simulink model "simscape_trial_simplified"  (R2020a)
settings: Solver=VariableStepAuto  StartTime=0.0  StopTime=tf  FixedStep=0.001  MaxStep=.0001  RelTol=1e-3  AbsTol=1e-3
PreLoadFcn:
  | simscape_trial_simplified_script
undefined symbols (not defined in the file): DC, numberNozzles
libraries: nesl_utility x7, fl_lib x6, SimscapeFluids_lib x6, sh_lib x2
settings Model: Creator=kenny  LastModifiedBy=voncken
settings SolverCC: AutoScaleAbsTol=off
settings DebuggingCC: SymbolicDimsDataTypeCodeGenerationDiagnostic=none
settings SFSimCC: CustomCodeUndefinedFunction=UseInterfaceOnly
settings SimscapeCC: SimscapeLogType=all  SimscapeLogSimulationStatistics=on  SimscapeLogLimitData=off  SimscapeLogDataHistory=10000

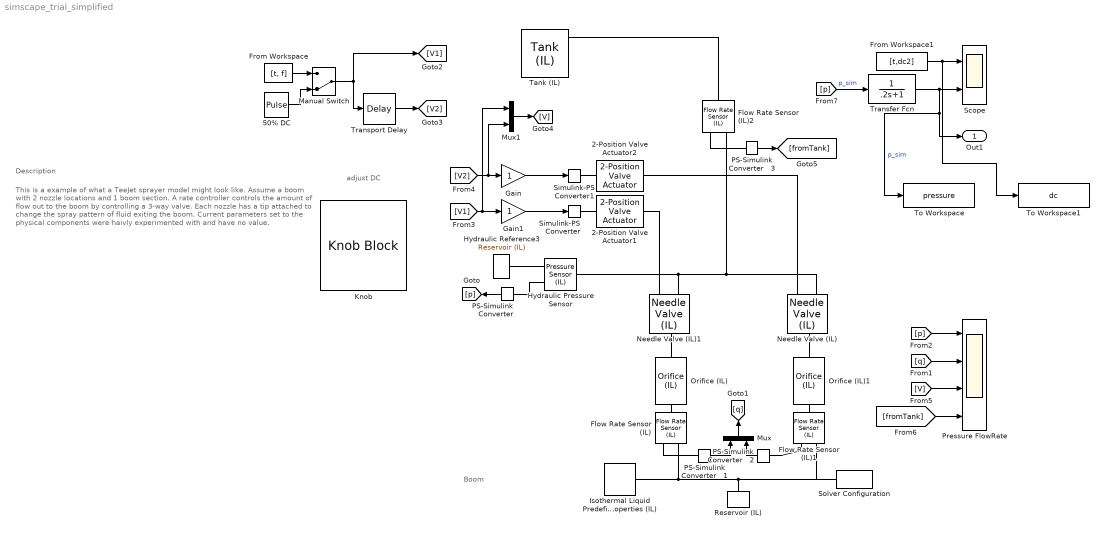
== system simscape_trial_simplified ==
  note: adjust DC
  note: Boom
  note: Description
  note: This is a example of what a TeeJet sprayer model might look like. Assume a boom with 2 nozzle locations and 1 boom section. A rate controller controls the amount of flow out to the boom by controlling a 3-way valve. Each nozzle has a tip attached to change the spray pattern of fluid exiting the boom.
      | Current parameters set to the physical components were haivly experimented with and have no value.
  2-Position Valve Actuator1 : sh_lib/Valves/Valve Actuators/2-Position Valve Actuator  stroke=h_MAX m  t_on=0.002 s  t_off=0.002 s  act_signal=12  init_position=0  act_orientation=1
      settings: SourceProductBaseCode=SH  InternalSimscapePortConfiguration="{\"Bottom\":[],\"Left\":[{\"id\":\"C\",\"label\":\"\",\"type\":\"input\"}],\"Right\":[{\"id\":\"P\",\"label\":\"\",\"type\":\"output\"}],\"Top\":[]}"
  2-Position Valve Actuator2 : sh_lib/Valves/Valve Actuators/2-Position Valve Actuator  stroke=h_MAX m  t_on=0.002 s  t_off=0.002 s  act_signal=12  init_position=0  act_orientation=1
      settings: SourceProductBaseCode=SH  InternalSimscapePortConfiguration="{\"Bottom\":[],\"Left\":[{\"id\":\"C\",\"label\":\"\",\"type\":\"input\"}],\"Right\":[{\"id\":\"P\",\"label\":\"\",\"type\":\"output\"}],\"Top\":[]}"
  "50% DC  " : DiscretePulseGenerator  PulseType=Time based  Amplitude=12  Period=.05  PulseWidth=DC
  Flow Rate Sensor (IL) : fl_lib/Isothermal Liquid/Sensors/Flow Rate Sensor (IL)  sensor_type=foundation.enum.mass_volumetric_sensor.volumetric
      settings: SourceProductBaseCode=SS  InternalSimscapePortConfiguration="{\"Bottom\":[],\"Left\":[{\"id\":\"A\",\"label\":\"A\",\"type\":\"foundation.isothermal_liquid.isothermal_liquid\"}],\"Right\":[{\"id\":\"B\",\"label\":\"B\",\"type\":\"foundation.isothermal_liquid.isothermal_liquid\"},{\"id\":\"V\",\"label\":\"V\",\"type\":\"output\"}],\"Top\":[]}"
  Flow Rate Sensor (IL)1 : fl_lib/Isothermal Liquid/Sensors/Flow Rate Sensor (IL)  sensor_type=foundation.enum.mass_volumetric_sensor.volumetric
      settings: SourceProductBaseCode=SS  InternalSimscapePortConfiguration="{\"Bottom\":[],\"Left\":[{\"id\":\"A\",\"label\":\"A\",\"type\":\"foundation.isothermal_liquid.isothermal_liquid\"}],\"Right\":[{\"id\":\"B\",\"label\":\"B\",\"type\":\"foundation.isothermal_liquid.isothermal_liquid\"},{\"id\":\"V\",\"label\":\"V\",\"type\":\"output\"}],\"Top\":[]}"
  Flow Rate Sensor (IL)2 : fl_lib/Isothermal Liquid/Sensors/Flow Rate Sensor (IL)  sensor_type=foundation.enum.mass_volumetric_sensor.volumetric
      settings: SourceProductBaseCode=SS  InternalSimscapePortConfiguration="{\"Bottom\":[],\"Left\":[{\"id\":\"A\",\"label\":\"A\",\"type\":\"foundation.isothermal_liquid.isothermal_liquid\"}],\"Right\":[{\"id\":\"B\",\"label\":\"B\",\"type\":\"foundation.isothermal_liquid.isothermal_liquid\"},{\"id\":\"V\",\"label\":\"V\",\"type\":\"output\"}],\"Top\":[]}"
  From Workspace : FromWorkspace  VariableName=[t, f]
  From Workspace1 : FromWorkspace  VariableName=[t,dc2]  SampleTime=-1
  Gain : Gain
  Gain1 : Gain
  Hydraulic Pressure Sensor : fl_lib/Isothermal Liquid/Sensors/Pressure Sensor (IL)  pressure_measure=foundation.enum.pressure_measure.difference
      settings: SourceProductBaseCode=SS  InternalSimscapePortConfiguration="{\"Bottom\":[],\"Left\":[{\"id\":\"A\",\"label\":\"A\",\"type\":\"foundation.isothermal_liquid.isothermal_liquid\"}],\"Right\":[{\"id\":\"B\",\"label\":\"B\",\"type\":\"foundation.isothermal_liquid.isothermal_liquid\"},{\"id\":\"P\",\"label\":\"P\",\"type\":\"output\"}],\"Top\":[]}"
  Hydraulic Reference3 : fl_lib/Isothermal Liquid/Elements/Reservoir (IL)  reservoir_type=foundation.enum.constant_controlled.constant  pressure_spec=foundation.enum.pressure_spec.atmospheric  reservoir_pressure=0.101325 MPa
      settings: SourceProductBaseCode=SS
  Isothermal Liquid Predefined Properties (IL) : SimscapeFluids_lib/Isothermal Liquid/Utilities/Isothermal Liquid Predefined Properties (IL)  fluid_list=fluids.isothermal_liquid.utilities.enum.isothermal_liquid_fluid_list.water  concentration_param_EG=fluids.isothermal_liquid.utilities.enum.isothermal_liquid_concentration.volume_fraction  concentration_param_PG=fluids.isothermal_liquid.utilities.enum.isothermal_liquid_concentration.volume_fraction  c_mass_SW=3.5e-3  c_mass_EG=0.1  c_mass_PG=0.1  c_mass_GL=0.1  c_vol_EG=0.1  c_vol_PG=0.1  beta_L_atm_EG=2.1791 GPa  beta_L_atm_PG=2.1791 GPa  beta_L_atm_GL=2.1791 GPa  p_min_EG=0.01 MPa  p_min_PG=0.01 MPa  p_min_GL=0.01 MPa  T=293.15 K  air_fraction=0  polytropic_index=1.0  rho_g_atm=1.225 kg/m^3  air_dissolution_model=simscape.enum.onoff.off  p_crit=3 MPa  derate_coeff=1  p_atm=0.101325 MPa
      settings: SourceProductBaseCode=SH  InternalSimscapePortConfiguration="{\"Bottom\":[],\"Left\":[],\"Right\":[{\"id\":\"A\",\"label\":\"\",\"type\":\"foundation.isothermal_liquid.isothermal_liquid\"}],\"Top\":[]}"
  Knob : KnobBlock  TickInterval=10
  Manual Switch : ManualSwitch  CurrentSetting=0
  Mux : Mux  Inputs=2
  Mux1 : Mux  Inputs=2
  Needle Valve (IL) : SimscapeFluids_lib/Isothermal Liquid/Valves & Orifices/Flow Control Valves/Needle Valve (IL)  diam_orifice=5e-3 m  cone_angle=90 deg  S_min=0 m  area_leak=1e-10*numberNozzles m^2  area=inf m^2  Cd=0.64  Re_c=150  pressure_recovery=simscape.enum.onoff.off  mdot_A_specify=off  mdot_A_priority=None  mdot_A=0 kg/s  mdot_A_nominal_specify=off  mdot_A_nominal_unit=kg/s  mdot_A_nominal_value=1  mdot_B_specify=off  mdot_B_priority=None  mdot_B=0 kg/s  mdot_B_nominal_specify=off  mdot_B_nominal_unit=kg/s  mdot_B_nominal_value=1
      settings: SourceProductBaseCode=SH  InternalSimscapePortConfiguration="{\"Bottom\":[],\"Left\":[{\"id\":\"A\",\"label\":\"A\",\"type\":\"foundation.isothermal_liquid.isothermal_liquid\"},{\"id\":\"S\",\"label\":\"S\",\"type\":\"input\"}],\"Right\":[{\"id\":\"B\",\"label\":\"B\",\"type\":\"foundation.isothermal_liquid.isothermal_liquid\"}],\"Top\":[]}"
  Needle Valve (IL)1 : SimscapeFluids_lib/Isothermal Liquid/Valves & Orifices/Flow Control Valves/Needle Valve (IL)  diam_orifice=d_0 m  cone_angle=theta rad  S_min=0 m  area_leak=1e-10*numberNozzles m^2  area=inf m^2  Cd=0.64  Re_c=150  pressure_recovery=simscape.enum.onoff.off  mdot_A_specify=off  mdot_A_priority=None  mdot_A=0 kg/s  mdot_A_nominal_specify=off  mdot_A_nominal_unit=kg/s  mdot_A_nominal_value=1  mdot_B_specify=off  mdot_B_priority=None  mdot_B=0 kg/s  mdot_B_nominal_specify=off  mdot_B_nominal_unit=kg/s  mdot_B_nominal_value=1
      settings: SourceProductBaseCode=SH  InternalSimscapePortConfiguration="{\"Bottom\":[],\"Left\":[{\"id\":\"A\",\"label\":\"A\",\"type\":\"foundation.isothermal_liquid.isothermal_liquid\"},{\"id\":\"S\",\"label\":\"S\",\"type\":\"input\"}],\"Right\":[{\"id\":\"B\",\"label\":\"B\",\"type\":\"foundation.isothermal_liquid.isothermal_liquid\"}],\"Top\":[]}"
  Orifice (IL) : SimscapeFluids_lib/Isothermal Liquid/Valves & Orifices/Orifices/Orifice (IL)  orifice_type=foundation.enum.constant_variable.constant  constant_orifice_spec=fluids.isothermal_liquid.valves_orifices.orifices.enum.constant_orifice_spec.table1D_volflow_pressure  variable_orifice_spec=fluids.isothermal_liquid.valves_orifices.orifices.enum.orifice_spec.linear  orifice_area_constant=1e-3 m^2  p_diff_TLU_constant=pressureDrop psi  vol_flow_TLU_constant=volFlowRate gpm  S_min=0 m  del_S=5e-3 m  open_orientation=fluids.isothermal_liquid.valves_orifices.orifices.enum.orifice_orientation.positive  area_max=1e-4 m^2  area_leak=1e-10 m^2  S_TLU=[0, .002, .004, .007, .017] m  orifice_area_TLU=[1e-09, 2.0352e-07, 4.0736e-05, .00011438, .00034356] m^2  area=inf m^2  Cd=0.64  Re_c=150  pressure_recovery=simscape.enum.onoff.off  S_vol_flow_TLU=[0, .002, .004, .007, .017] m  p_diff_TLU=[.3, .5, .7] MPa  vol_flow_TLU=1e-3 * [1.7e-05, 2e-05, 2.6e-05; .0035, .0045, .0053; .7, .9, 1.06; 1.96, 2.5, 3; 6, 7.7, 9.13] m^3/s  mdot_A_specify=off  mdot_A_priority=None  mdot_A=0 kg/s  mdot_A_nominal_specify=off  mdot_A_nominal_unit=kg/s  mdot_A_nominal_value=1  mdot_B_specify=off  mdot_B_priority=None  mdot_B=0 kg/s  mdot_B_nominal_specify=off  mdot_B_nominal_unit=kg/s  mdot_B_nominal_value=1
      settings: SourceProductBaseCode=SH  InternalSimscapePortConfiguration="{\"Bottom\":[],\"Left\":[{\"id\":\"A\",\"label\":\"A\",\"type\":\"foundation.isothermal_liquid.isothermal_liquid\"}],\"Right\":[{\"id\":\"B\",\"label\":\"B\",\"type\":\"foundation.isothermal_liquid.isothermal_liquid\"}],\"Top\":[]}"
  Orifice (IL)1 : SimscapeFluids_lib/Isothermal Liquid/Valves & Orifices/Orifices/Orifice (IL)  orifice_type=foundation.enum.constant_variable.constant  constant_orifice_spec=fluids.isothermal_liquid.valves_orifices.orifices.enum.constant_orifice_spec.table1D_volflow_pressure  variable_orifice_spec=fluids.isothermal_liquid.valves_orifices.orifices.enum.orifice_spec.linear  orifice_area_constant=1e-3 m^2  p_diff_TLU_constant=pressureDrop psi  vol_flow_TLU_constant=volFlowRate gpm  S_min=0 m  del_S=5e-3 m  open_orientation=fluids.isothermal_liquid.valves_orifices.orifices.enum.orifice_orientation.positive  area_max=1e-4 m^2  area_leak=1e-10 m^2  S_TLU=[0, .002, .004, .007, .017] m  orifice_area_TLU=[1e-09, 2.0352e-07, 4.0736e-05, .00011438, .00034356] m^2  area=inf m^2  Cd=0.64  Re_c=150  pressure_recovery=simscape.enum.onoff.off  S_vol_flow_TLU=[0, .002, .004, .007, .017] m  p_diff_TLU=[.3, .5, .7] MPa  vol_flow_TLU=1e-3 * [1.7e-05, 2e-05, 2.6e-05; .0035, .0045, .0053; .7, .9, 1.06; 1.96, 2.5, 3; 6, 7.7, 9.13] m^3/s  mdot_A_specify=off  mdot_A_priority=None  mdot_A=0 kg/s  mdot_A_nominal_specify=off  mdot_A_nominal_unit=kg/s  mdot_A_nominal_value=1  mdot_B_specify=off  mdot_B_priority=None  mdot_B=0 kg/s  mdot_B_nominal_specify=off  mdot_B_nominal_unit=kg/s  mdot_B_nominal_value=1
      settings: SourceProductBaseCode=SH  InternalSimscapePortConfiguration="{\"Bottom\":[],\"Left\":[{\"id\":\"A\",\"label\":\"A\",\"type\":\"foundation.isothermal_liquid.isothermal_liquid\"}],\"Right\":[{\"id\":\"B\",\"label\":\"B\",\"type\":\"foundation.isothermal_liquid.isothermal_liquid\"}],\"Top\":[]}"
  "PS-Simulink Converter   " : nesl_utility/PS-Simulink Converter  PhysicalDomain=network_engine_domain  SubClassName=ps_output  LeftPortType=input  RightPortType=output  PseudoPeriodic=off  Frequencies=[]  Unit=bar  AffineConversion=off
      settings: SourceProductBaseCode=MT,SS
  PS-Simulink Converter   1 : nesl_utility/PS-Simulink Converter  PhysicalDomain=network_engine_domain  SubClassName=ps_output  LeftPortType=input  RightPortType=output  PseudoPeriodic=off  Frequencies=[]  Unit=gpm  AffineConversion=off
      settings: SourceProductBaseCode=MT,SS
  PS-Simulink Converter   2 : nesl_utility/PS-Simulink Converter  PhysicalDomain=network_engine_domain  SubClassName=ps_output  LeftPortType=input  RightPortType=output  PseudoPeriodic=off  Frequencies=[]  Unit=gpm  AffineConversion=off
      settings: SourceProductBaseCode=MT,SS
  PS-Simulink Converter   3 : nesl_utility/PS-Simulink Converter  PhysicalDomain=network_engine_domain  SubClassName=ps_output  LeftPortType=input  RightPortType=output  PseudoPeriodic=off  Frequencies=[]  Unit=gpm  AffineConversion=off
      settings: SourceProductBaseCode=MT,SS
  Pressure FlowRate : Scope  NumInputPorts=4
  Reservoir (IL) : fl_lib/Isothermal Liquid/Elements/Reservoir (IL)  reservoir_type=foundation.enum.constant_controlled.constant  pressure_spec=foundation.enum.pressure_spec.atmospheric  reservoir_pressure=0.101325 MPa
      settings: SourceProductBaseCode=SS
  Scope : Scope  NumInputPorts=2
  Simulink-PS Converter : nesl_utility/Simulink-PS Converter  PhysicalDomain=network_engine_domain  SubClassName=ps_input  LeftPortType=input  RightPortType=output  PseudoPeriodic=off  Frequencies=[]  NoiseDistribution=none  NoiseParameters=[]  Unit=1  AffineConversion=off  FilteringAndDerivatives=provide  SimscapeFilterOrder=1  InputFilterTimeConstant=0.001  UdotUserProvided=0
  Simulink-PS Converter1 : nesl_utility/Simulink-PS Converter  PhysicalDomain=network_engine_domain  SubClassName=ps_input  LeftPortType=input  RightPortType=output  PseudoPeriodic=off  Frequencies=[]  NoiseDistribution=none  NoiseParameters=[]  Unit=1  AffineConversion=off  FilteringAndDerivatives=provide  SimscapeFilterOrder=1  InputFilterTimeConstant=0.001  UdotUserProvided=0
  Solver Configuration : nesl_utility/Solver Configuration  PhysicalDomain=network_engine_domain  SubClassName=solver  LeftPortType=input  RightPortType=generic  Tones=[]  Harmonics=[]  SimulateNoise=off  Profile=off  UseLocalSampling=off  EnableSwitchedLinearOptims=on  FrequencyDomain=off  UseCCode=off  RelTol=0.001  AbsTol=1e-06  MinStep=1e-09  ToWorkspace=off  RevertToSquareIcSolve=off  NumHomotopyIterations=100  PhasorMode=off  PhasorModeNumHarmonics=1  DoDC=off  ResidualTolerance=1e-09  UseLocalSolver=off  LocalSolverChoice=NE_TRAPEZOIDAL_ADVANCER  LocalSolverSampleTime=0.001  DoFixedCost=off  MaxNonlinIter=3  MaxModeIter=2  LinearAlgebra=auto  EquationFormulation=NE_TIME_EF  DelaysMemoryBudget=1024  AutomaticFiltering=on  FilteringTimeConstant=0.001  PartitionStorageMethod=AS_NEEDED  PartitionMemoryBudget=1024  PartitionMethod=ROBUST
      settings: SourceProductBaseCode=MT,SS
  Tank (IL) : SimscapeFluids_lib/Isothermal Liquid/Tanks & Accumulators/Tank (IL)  num_inlet=fluids.isothermal_liquid.tanks_accumulators.enum.num_inlet.one  pressure_spec=foundation.enum.pressure_spec.atmospheric  tank_pressure=0.101325 MPa  volume_spec=fluids.isothermal_liquid.tanks_accumulators.enum.tank_volume_spec.constant  tank_area=.8 m^2  level_TLU=[0, 3, 5] m  volume_TLU=[0, 4, 6] m^3  inlet_height_A=1e-3 m  inlet_area_A=pi*0.02^2/4 m^2  loss_coeff_A=1.2  inlet_height_AB=[.1, 0] m  inlet_area_AB=[.01, .01] m^2  loss_coeff_AB=[1.2, 1.2]  inlet_height_ABC=[.1, .05, 0] m  inlet_area_ABC=[.01, .01, .01] m^2  loss_coeff_ABC=[1.2, 1.2, 1.2]  inlet_height_ABCD=linspace(0.1, 0, 4) m  inlet_area_ABCD=0.01 * ones(1, 4) m^2  loss_coeff_ABCD=1.2 * ones(1, 4)  inlet_height_ABCDE=linspace(0.1, 0, 5) m  inlet_area_ABCDE=0.01 * ones(1, 5) m^2  loss_coeff_ABCDE=1.2 * ones(1, 5)  inlet_height_ABCDEF=linspace(0.1, 0, 6) m  inlet_area_ABCDEF=0.01 * ones(1, 6) m^2  loss_coeff_ABCDEF=1.2 * ones(1, 6)  level_check=simscape.enum.assert.action.error  capacity_check=simscape.enum.assert.action.none  max_capacity=10 m^3  g=9.81 m/s^2  level_specify=on  level_priority=High  level=2.8*12 m  level_nominal_specify=off  level_nominal_unit=m  level_nominal_value=1  volume_specify=off  volume_priority=None  volume=5 m^3  volume_nominal_specify=off  volume_nominal_unit=m^3  volume_nominal_value=1  mass_specify=off  mass_priority=None  mass=5e+3 kg  mass_nominal_specify=off  mass_nominal_unit=kg  mass_nominal_value=1
      settings: SourceProductBaseCode=SH  InternalSimscapePortConfiguration="{\"Bottom\":[],\"Left\":[{\"id\":\"A\",\"label\":\"A\",\"type\":\"foundation.isothermal_liquid.isothermal_liquid\"}],\"Right\":[],\"Top\":[{\"id\":\"V\",\"label\":\"V\",\"type\":\"output\"},{\"id\":\"L\",\"label\":\"L\",\"type\":\"output\"}]}"
  To Workspace : ToWorkspace  VariableName=pressure  SaveFormat=Timeseries  SampleTime=-1
  To Workspace1 : ToWorkspace  VariableName=dc  SaveFormat=Timeseries  SampleTime=-1
  Transfer Fcn : TransferFcn  Denominator=[.2 1]
  Transport Delay : TransportDelay  DelayTime=.025
  Out1 : Outport
  wires:
  "PS-Simulink Converter   "/1 -> [p]
  PS-Simulink Converter   1/1 -> Mux/1
  PS-Simulink Converter   2/1 -> Mux/2
  Mux/1 -> [q]
  [p] -> Pressure FlowRate/1
  [q] -> Pressure FlowRate/2
  Transport Delay/1 -> [V2]
  [V1] -> Mux1/1, Gain1/1
  [V2] -> Mux1/2, Gain/1
  Gain/1 -> Simulink-PS Converter1/1
  Gain1/1 -> Simulink-PS Converter/1
  Mux1/1 -> [V]
  [V] -> Pressure FlowRate/3
  PS-Simulink Converter   3/1 -> [fromTank]
  [fromTank] -> Pressure FlowRate/4
  From Workspace/1 -> Manual Switch/1
  "50% DC  "/1 -> Manual Switch/2
  Manual Switch/1 -> [V1], Transport Delay/1
  From Workspace1/1 -> To Workspace1/1, Scope/1
  [p] -> Transfer Fcn/1  "p_sim"
  Transfer Fcn/1 -> To Workspace/1, Out1/1, Scope/2  "p_sim"
  connections:
  Hydraulic Pressure Sensor/LConn1 -- Needle Valve (IL)/LConn1 -- Flow Rate Sensor (IL)2/RConn1 -- Needle Valve (IL)1/LConn1
  Hydraulic Pressure Sensor/RConn2 -- "PS-Simulink Converter   "/LConn1
  Hydraulic Pressure Sensor/RConn1 -- Hydraulic Reference3/LConn1
  Orifice (IL)/LConn1 -- Needle Valve (IL)1/RConn1
  Orifice (IL)1/LConn1 -- Needle Valve (IL)/RConn1
  Isothermal Liquid Predefined Properties (IL)/RConn1 -- Flow Rate Sensor (IL)/RConn1 -- Flow Rate Sensor (IL)1/RConn1 -- Solver Configuration/RConn1 -- Reservoir (IL)/LConn1
  Flow Rate Sensor (IL)/LConn1 -- Orifice (IL)/RConn1
  Flow Rate Sensor (IL)1/LConn1 -- Orifice (IL)1/RConn1
  Flow Rate Sensor (IL)/RConn2 -- PS-Simulink Converter   1/LConn1
  PS-Simulink Converter   2/LConn1 -- Flow Rate Sensor (IL)1/RConn2
  Simulink-PS Converter/RConn1 -- 2-Position Valve Actuator1/LConn1
  Simulink-PS Converter1/RConn1 -- 2-Position Valve Actuator2/LConn1
  2-Position Valve Actuator1/RConn1 -- Needle Valve (IL)1/LConn2
  2-Position Valve Actuator2/RConn1 -- Needle Valve (IL)/LConn2
  Flow Rate Sensor (IL)2/RConn2 -- PS-Simulink Converter   3/LConn1
  Flow Rate Sensor (IL)2/LConn1 -- Tank (IL)/LConn1
